simulink model "ControleEEcanalI"  (R2022b)
settings: Solver=ode45  StartTime=0.0  StopTime=30  RelTol=1e-7  EnableMultiTasking=on
values from neighbouring files (symbols this model uses):
  K = acker(A,B,p)    [PrObsPertContinuoRed.m]    (also in PrPara2nl_PI.m = acker(Aa,Ba,[p,p,p]); TestesEE.m = acker(A,B,[p,p,p]); TestesEEcanalI.m = acker(A,B,[p,-.6-1.0198i,-.6+1.0198i]); TestesEEobsPert.m = acker(A,B,[p,-.6-1.0198i,-.6+1.0198i]))
  Ki = -K(3)    [PrPara2nl_PI.m]    (also in TestesEEcanalI.m = -Ka(4),K=Ka(1:3),; para2nl_PI.m)
  L = L'    [PrObsPertContinuoRed.m]    (also in PrPara2nl_PI.m; TestesEE.m; TestesEEcanalI.m; TestesEEobsPert.m)
  Lc = L(4)    [TestesEEcanalI.m]    (also in TestesEEobsPert.m)
  Nb = gf.den{1}(1,2)/gf.num{1}(1,2)    [PrObsPertContinuoRed.m]    (also in PrPara2nl_PI.m = gf.den{1}(1,3)/gf.num{1}(1,3); TestesEE.m = gf.den{1}(1,4)/gf.num{1}(1,4); TestesEEcanalI.m = gf.den{1}(1,4)/gf.num{1}(1,4); TestesEEobsPert.m = gf.den{1}(1,4)/gf.num{1}(1,4))
settings Model: Creator=Adolfo  LastModifiedBy=adolfo
settings SolverCC: AlgebraicLoopSolver=TrustRegion
settings DataIOCC: LimitDataPoints=on  SaveFormat=Array  SignalLoggingSaveFormat=ModelDataLogs  ReturnWorkspaceOutputs=off
settings OptimizationCC: ExpressionDepthLimit=2147483647  InitFltsAndDblsToZero=on  LifeSpan=inf
settings DebuggingCC: SaveWithParameterizedLinksMsg=none  UnderspecifiedInitializationDetection=Classic  MergeDetectMultiDrivingBlocksExec=none  SignalResolutionControl=TryResolveAllWithWarning  MultiTaskDSMMsg=warning  MultiTaskCondExecSysMsg=none  FcnCallInpInsideContextMsg=warning  UnconnectedInputMsg=warning  UnconnectedOutputMsg=warning  UnconnectedLineMsg=warning  StateNameClashWarn=warning  SFUnexpectedBacktrackingDiag=warning  SFNoUnconditionalDefaultTransitionDiag=warning  SFExecutionAtInitializationDiag=none  SFMachineParentedDataDiag=warning  ArithmeticOperatorsInVariantConditions=warning
settings HardwareCC: ProdBitPerPointer=32  ProdBitPerSizeT=32  ProdBitPerPtrDiffT=32  ProdLargestAtomicFloat=None  ProdIntDivRoundTo=Undefined  ProdEndianess=Unspecified  ProdWordSize=32  ProdHWDeviceType=32-bit Generic
settings ModelReferenceCC: EnableRefExpFcnMdlSchedulingChecks=on  PropagateSignalLabelsOutOfModel=off
settings SFSimCC: SimUseLocalCustomCode=off  CustomCodeUndefinedFunction=UseInterfaceOnly
settings RTWCC: RTWUseLocalCustomCode=off
settings CodeAppCC: StateflowObjectComments=on
settings GRTTargetCC: TargetFcnLib=ansi_tfl_tmw.mat  TargetLangStandard=C89/C90 (ANSI)  CombineOutputUpdateFcns=off  GRTInterface=on
settings ConfigComp: CovMetricSettings=dw  CovSaveCumulativeToWorkspaceVar=on  CovSaveSingleToWorkspaceVar=on  CovExternalEMLEnable=off  CovSFcnEnable=off

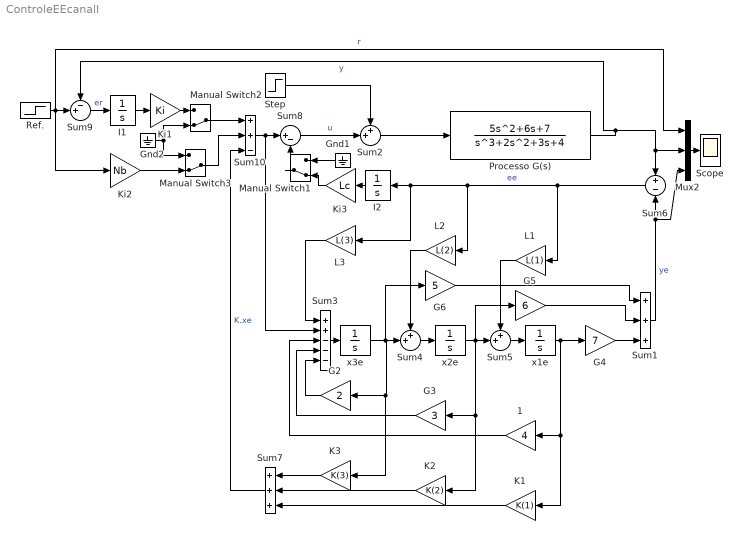
== system ControleEEcanalI ==
  1 : Gain  Gain=4
  G2 : Gain  Gain=2
  G3 : Gain  Gain=3
  G4 : Gain  Gain=7
  G5 : Gain  Gain=6
  G6 : Gain  Gain=5
  Gnd1 : Ground
  Gnd2 : Ground
  I1 : Integrator
  I2 : Integrator
  K1 : Gain  Gain=K(1)
  K2 : Gain  Gain=K(2)
  K3 : Gain  Gain=K(3)
  Ki1 : Gain  Gain=Ki
  Ki2 : Gain  Gain=Nb
  Ki3 : Gain  Gain=Lc
  L1 : Gain  Gain=L(1)
  L2 : Gain  Gain=L(2)
  L3 : Gain  Gain=L(3)
  Manual Switch1 : ManualSwitch  CurrentSetting=0
  Manual Switch2 : ManualSwitch  CurrentSetting=0
  Manual Switch3 : ManualSwitch  CurrentSetting=0
  Mux2 : Mux  Inputs=3
  Processo G(s) : TransferFcn  Numerator=[5 6 7]  Denominator=[1 2 3 4]
  Ref. : Step  Time=0  SampleTime=0
  Scope : Scope
  Step : Step  Time=10  SampleTime=0
  Sum1 : Sum  Inputs=+++
  Sum10 : Sum  Inputs=++-
  Sum2 : Sum  Inputs=++|
  Sum3 : Sum  Inputs=++---
  Sum4 : Sum  Inputs=++|
  Sum5 : Sum  Inputs=++|
  Sum6 : Sum  Inputs=+-
  Sum7 : Sum  Inputs=+++
  Sum8 : Sum  Inputs=|+-
  Sum9 : Sum  Inputs=-+|
  x1e : Integrator
  x2e : Integrator
  x3e : Integrator
  wires:
  Ref./1 -> Ki2/1, Mux2/1, Sum9/2  "r"
  Mux2/1 -> Scope/1
  x3e/1 -> G6/1, Sum4/2, G2/1, K3/1
  x2e/1 -> G3/1, K2/1, G5/1, Sum5/2
  Sum3/1 -> x3e/1
  G2/1 -> Sum3/5
  G3/1 -> Sum3/4
  x1e/1 -> G4/1, K1/1, 1/1
  1/1 -> Sum3/3
  G4/1 -> Sum1/3
  Processo G(s)/1 -> Sum6/1, Mux2/2, Sum9/1  "y"
  Sum1/1 -> Sum6/2, Mux2/3  "ye"
  Sum4/1 -> x2e/1
  Sum5/1 -> x1e/1
  Sum6/1 -> L2/1, L3/1, I2/1, L1/1  "ee"
  L3/1 -> Sum3/1
  L2/1 -> Sum4/1
  L1/1 -> Sum5/1
  Step/1 -> Sum2/1
  K3/1 -> Sum7/1
  K2/1 -> Sum7/2
  K1/1 -> Sum7/3
  Sum10/1 -> Sum3/2, Sum8/1
  I2/1 -> Ki3/1
  Sum2/1 -> Processo G(s)/1
  I1/1 -> Ki1/1
  Sum7/1 -> Sum10/3  "K.xe"
  Sum9/1 -> I1/1  "er"
  Manual Switch2/1 -> Sum10/1
  Ki1/1 -> Manual Switch2/1
  Manual Switch1/1 -> Sum8/2
  Manual Switch3/1 -> Sum10/2
  Sum8/1 -> Sum2/2  "u"
  G6/1 -> Sum1/1
  G5/1 -> Sum1/2
  Gnd2/1 -> Manual Switch3/1, Manual Switch2/2
  Ki2/1 -> Manual Switch3/2
  Ki3/1 -> Manual Switch1/2
  Gnd1/1 -> Manual Switch1/1
